simulink model "controller_ver"  (R2020b)
settings: Solver=ode45  StartTime=0.0  StopTime=10.0  MaxStep=0.01  RelTol=1e-3
undefined symbols (not defined in the file): K_d, K_p, params, r_des
settings Model: Creator=Danil  LastModifiedBy=Danil

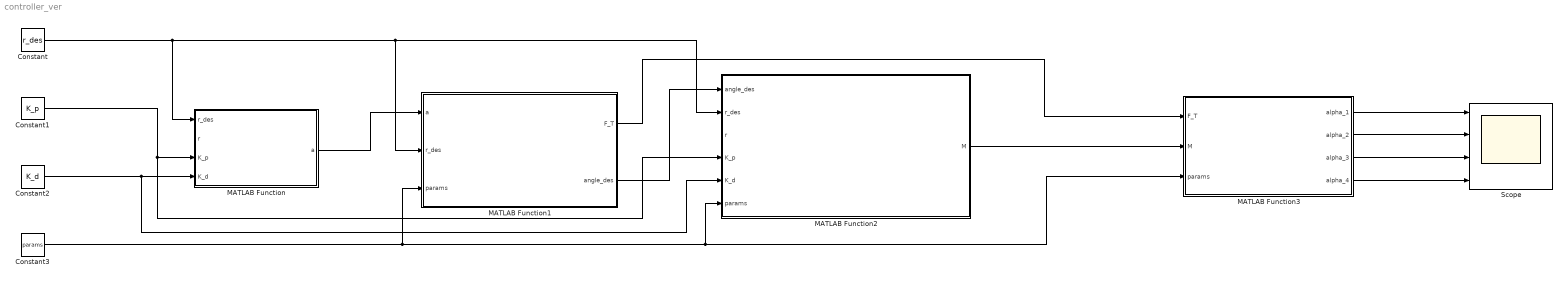
== system controller_ver ==
  Constant : Constant  Value=r_des  OutDataTypeStr=Bus: r_des_bus
  Constant1 : Constant  Value=K_p  OutDataTypeStr=Bus: K_p_bus
  Constant2 : Constant  Value=K_d  OutDataTypeStr=Bus: K_d_bus
  Constant3 : Constant  Value=params  OutDataTypeStr=Bus: params_bus
  MATLAB Function : MATLAB Function  TreatAsAtomicUnit=on
  MATLAB Function1 : MATLAB Function  TreatAsAtomicUnit=on
  MATLAB Function2 : MATLAB Function  TreatAsAtomicUnit=on
  MATLAB Function3 : MATLAB Function  TreatAsAtomicUnit=on
  Scope : Scope  NumInputPorts=4
  wires:
  MATLAB Function/1(a) -> MATLAB Function1/1(a)
  MATLAB Function1/2(angle_des) -> MATLAB Function2/1(angle_des)
  MATLAB Function2/1(M) -> MATLAB Function3/2(M)
  MATLAB Function1/1(F_T) -> MATLAB Function3/1(F_T)
  Constant/1 -> MATLAB Function/1(r_des), MATLAB Function1/2(r_des), MATLAB Function2/2(r_des)
  Constant1/1 -> MATLAB Function/3(K_p), MATLAB Function2/4(K_p)
  Constant2/1 -> MATLAB Function/4(K_d), MATLAB Function2/5(K_d)
  Constant3/1 -> MATLAB Function1/3(params), MATLAB Function2/6(params), MATLAB Function3/3(params)
  MATLAB Function3/1(alpha_1) -> Scope/1
  MATLAB Function3/2(alpha_2) -> Scope/2
  MATLAB Function3/3(alpha_3) -> Scope/3
  MATLAB Function3/4(alpha_4) -> Scope/4

== matlab function controller_ver/MATLAB Function1 ==
  data: F_T output; angle_des output; a input; r_des input; params input
function [F_T, angle_des] = fcn(a, r_des, params)

F_T = params.m * (a.z_ddot + params.g);

fi_des = (1 / params.g) * (a.x_ddot * sin(r_des.psi) - a.y_ddot * cos(r_des.psi));
theta_des = (1 / params.g) * (a.x_ddot * cos(r_des.psi) + a.y_ddot * sin(r_des.psi));
psi_des = r_des.psi;

angle_des.fi_des = fi_des;
angle_des.theta_des = theta_des;
angle_des.psi_des = psi_des;

== matlab function controller_ver/MATLAB Function ==
  data: r_des input; a output; r input; K_p input; K_d input
function a  = fcn(r_des, r, K_p, K_d)

x_ddot = r_des.x_ddot + K_d.x * (r_des.x_dot - r.x_dot) + K_p.x * (r_des.x - r.x);
y_ddot = r_des.y_ddot + K_d.y * (r_des.y_dot - r.y_dot) + K_p.y * (r_des.y - r.y);
z_ddot = r_des.z_ddot + K_d.z * (r_des.z_dot - r.z_dot) + K_p.z * (r_des.z - r.z);

a.x_ddot = x_ddot;
a.y_ddot = y_ddot;
a.z_ddot = z_ddot;

== matlab function controller_ver/MATLAB Function2 ==
  data: angle_des input; r_des input; r input; M output; K_p input; K_d input; params input
function M = fcn(angle_des, r_des, r, K_p, K_d, params)

M_x = (params.J_xx / params.L_x) * (r_des.fi_ddot + K_d.fi * (r_des.fi_dot - r.fi_dot) + K_p.fi * (angle_des.fi_des - r.fi));
M_y = (params.J_yy / params.L_y) * (r_des.theta_ddot + K_d.theta * (r_des.theta_dot - r.theta_dot) + K_p.theta * (angle_des.theta_des - r.theta));
M_z = (params.J_zz / params.L_z) * (r_des.psi_ddot + K_d.psi * (r_des.psi_dot - r.psi_dot) + K_p.psi * (angle_des.psi_des - r.psi));

M.M_x = M_x;
M.M_y = M_y;
M.M_z = M_z;

== matlab function controller_ver/MATLAB Function3 ==
  data: F_T input; alpha_1 output; M input; params input; alpha_2 output; alpha_3 output; alpha_4 output
function [alpha_1, alpha_2, alpha_3, alpha_4] = fcn(F_T, M, params)

alpha_1 = (1 / (4 * params.k_Y)) * (F_T + M.M_x + M.M_y + M.M_z) - 7;
alpha_2 = (1 / (4 * params.k_Y)) * (F_T + M.M_x - M.M_y - M.M_z);
alpha_3 = (1 / (4 * params.k_Y)) * (F_T - M.M_x + M.M_y - M.M_z) - 7;
alpha_4 = (1 / (4 * params.k_Y)) * (F_T - M.M_x - M.M_y + M.M_z);
